simulink model "SimulinkExport"  (R2024b)
settings: Solver=FixedStepDiscrete  StartTime=0.0  StopTime=20  FixedStep=0.01  MaxStep=0.001  RelTol=1e-3
settings Model: Creator=Green Crane Testbed  LastModifiedBy=Green Crane Testbed
settings ConfigComp: PLC_TargetIDE=plcopen  PLC_MultiTBSigbuilderTimeRange=off  PLC_FoldFBCallOutputVar=off  PLC_RemoveUnusedSSMethodCallArguments=off  PLC_UseCallOutputArgSyntax=off  PLC_EnableUnsignedAndDoubleTypes=off  PLC_EnableUDTSplitting=off  PLC_MaxFieldsInUDT=500  PLC_InlineEnumCastFunction=off

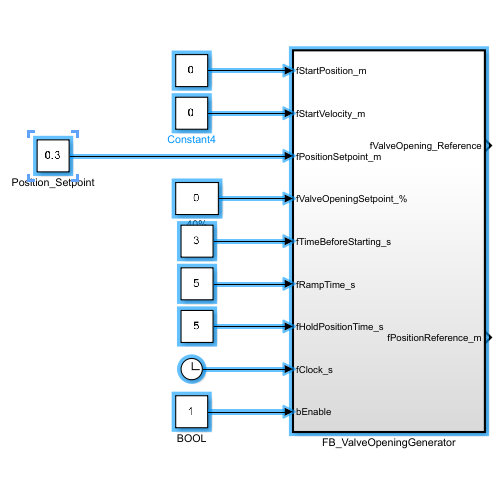
[thumbnail: Simulink's stored preview of the top-level diagram]
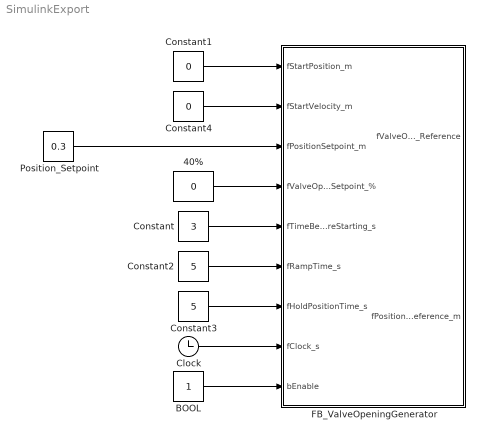
== system SimulinkExport ==
  40% : Constant  Value=0
  BOOL : Constant  OutDataTypeStr=boolean
  Clock : Clock
  Constant : Constant  Value=3
  Constant1 : Constant  Value=0
  Constant2 : Constant  Value=5
  Constant3 : Constant  Value=5
  Constant4 : Constant  Value=0
  FB_ValveOpeningGenerator : Subsystem  TreatAsAtomicUnit=on  VariantControl=Ramp_Profile
  Position_Setpoint : Constant  Value=0.3
  wires:
  40%/1 -> FB_ValveOpeningGenerator/4(fValveOpeningSetpoint_%)
  BOOL/1 -> FB_ValveOpeningGenerator/9(bEnable)
  Constant4/1 -> FB_ValveOpeningGenerator/2(fStartVelocity_m)
  Constant1/1 -> FB_ValveOpeningGenerator/1(fStartPosition_m)
  Constant2/1 -> FB_ValveOpeningGenerator/6(fRampTime_s)
  Position_Setpoint/1 -> FB_ValveOpeningGenerator/3(fPositionSetpoint_m)
  Constant3/1 -> FB_ValveOpeningGenerator/7(fHoldPositionTime_s)
  Clock/1 -> FB_ValveOpeningGenerator/8(fClock_s)
  Constant/1 -> FB_ValveOpeningGenerator/5(fTimeBeforeStarting_s)

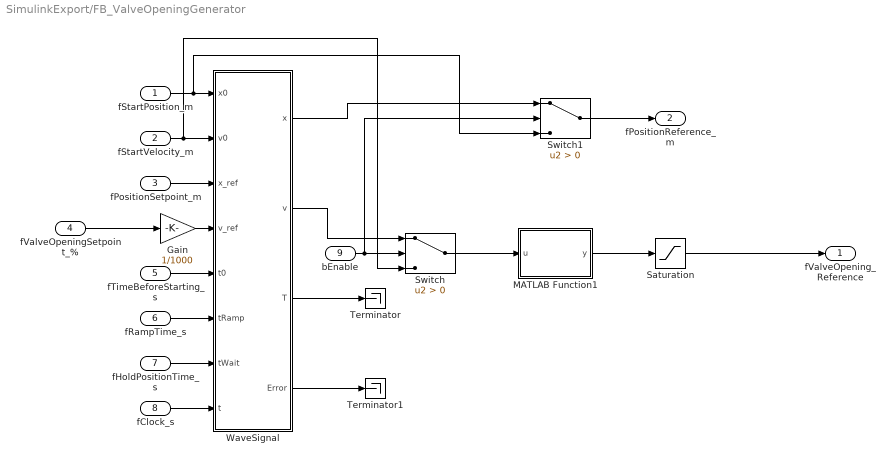
== system SimulinkExport/FB_ValveOpeningGenerator ==
  fStartPosition_m : Inport
  fStartVelocity_m : Inport  Port=2
  fPositionSetpoint_m : Inport  Port=3
  fValveOpeningSetpoint_% : Inport  Port=4
  fTimeBeforeStarting_s : Inport  Port=5
  fRampTime_s : Inport  Port=6
  fHoldPositionTime_s : Inport  Port=7
  fClock_s : Inport  Port=8
  bEnable : Inport  Port=9  OutDataTypeStr=boolean
  Gain : Gain  Gain=1/1000
  MATLAB Function1 : MATLAB Function  TreatAsAtomicUnit=on
  Saturation : Saturate
  Switch : Switch  Criteria=u2 > Threshold  SaturateOnIntegerOverflow=off  InputSameDT=off
  Switch1 : Switch  Criteria=u2 > Threshold  SaturateOnIntegerOverflow=off  InputSameDT=off
  Terminator : Terminator
  Terminator1 : Terminator
  WaveSignal : MATLAB Function  TreatAsAtomicUnit=on
  fValveOpening_Reference : Outport  VectorParamsAs1DForOutWhenUnconnected=off
  fPositionReference_m : Outport  Port=2  VectorParamsAs1DForOutWhenUnconnected=off
  wires:
  fClock_s/1 -> WaveSignal/8(t)
  fTimeBeforeStarting_s/1 -> WaveSignal/5(t0)
  fPositionSetpoint_m/1 -> WaveSignal/3(x_ref)
  fHoldPositionTime_s/1 -> WaveSignal/7(tWait)
  fValveOpeningSetpoint_%/1 -> Gain/1
  WaveSignal/3(T) -> Terminator/1
  fRampTime_s/1 -> WaveSignal/6(tRamp)
  WaveSignal/4(Error) -> Terminator1/1
  WaveSignal/2(v) -> Switch/1
  fStartPosition_m/1 -> Switch1/3, WaveSignal/1(x0)
  bEnable/1 -> Switch1/2, Switch/2
  WaveSignal/1(x) -> Switch1/1
  fStartVelocity_m/1 -> WaveSignal/2(v0), Switch/3
  MATLAB Function1/1(y) -> Saturation/1
  Switch/1 -> MATLAB Function1/1(u)
  Saturation/1 -> fValveOpening_Reference/1
  Switch1/1 -> fPositionReference_m/1
  Gain/1 -> WaveSignal/4(v_ref)

== matlab function SimulinkExport/FB_ValveOpeningGenerator/WaveSignal ==
  data: x0 input; v0 input; x_ref input; x output; v_ref input; t0 input; tRamp input; tWait input; v output; t input; T output; Error output double
function [x,v,T, Error] = fcn(x0,v0, x_ref,v_ref,t0,tRamp,tWait,t)
x_SP = x_ref - x0;
vs=v_ref;
slopeExt=v0-vs;
slopeRetr=-vs-v0;

as = vs/tRamp;
s_acc=(vs^2-v0^2)/as;

tHold=(x_SP-s_acc)/vs;

if tHold < 0
    Error = 1;
else
    Error = 0;
end

t1=tRamp;
t2=tHold;
t3=tRamp;
t4=tWait;
t5=t1;
t6=t2;
t7=t3;

x = x0;
x1 = x0 + v0*((t0+t1)-t0)-(slopeExt/t1)*((t0+t1)-t0)^2/2;
x2 = x1 + vs*((t0+t1+t2)-(t0+t1));
x4 = x_ref - v0*((t0+t1+t2+t3+t4+t5)-(t0+t1+t2+t3+t4))+(slopeRetr/t5)*((t0+t1+t2+t3+t4+t5)-(t0+t1+t2+t3+t4))^2/2;
x5 = x4-vs*((t0+t1+t2+t3+t4+t5+t6)-(t0+t1+t2+t3+t4+t5));

if Error == 1
    x = x0;
    v = v0;
elseif t>=0 && t<t0
    x = x0;
    v = v0;
elseif t>=t0 && t<(t0+t1)
    x = x0 + v0*(t-t0)-(slopeExt/t1)*(t-t0)^2/2;
    v = v0-(slopeExt/t1)*(t-t0);
elseif t>=(t0+t1) && t<(t0+t1+t2)
    x = x1 + vs*(t-(t0+t1));
    v = vs;
elseif t>=(t0+t1+t2) && t<(t0+t1+t2+t3)
    x = x2+vs*(t-(t0+t1+t2))+(slopeExt/t3)*(t-(t0+t1+t2))^2/2;
    v = vs+(slopeExt/t3)*(t-(t0+t1+t2));
elseif t>=(t0+t1+t2+t3) && t<(t0+t1+t2+t3+t4)
    x = x_ref;
    v = v0;
elseif t>=(t0+t1+t2+t3+t4) && t<(t0+t1+t2+t3+t4+t5)
    x = x_ref - v0*(t-(t0+t1+t2+t3+t4))+(slopeRetr/t5)*(t-(t0+t1+t2+t3+t4))^2/2;
    v = v0+(slopeRetr/t5)*(t-(t0+t1+t2+t3+t4));
elseif t>=(t0+t1+t2+t3+t4+t5) && t<(t0+t1+t2+t3+t4+t5+t6)
    x = x4-vs*(t-(t0+t1+t2+t3+t4+t5));
    v = -vs;
elseif t>=(t0+t1+t2+t3+t4+t5+t6) && t<(t0+t1+t2+t3+t4+t5+t6+t7)
    x = x5-vs*(t-(t0+t1+t2+t3+t4+t5+t6))-(slopeRetr/t3)*(t-(t0+t1+t2+t3+t4+t5+t6))^2/2;
    v = -vs-(slopeRetr/t3)*(t-(t0+t1+t2+t3+t4+t5+t6));
else
    x = x0;
    v = v0;
end

T = t0+t1+t2+t3+t4+t5+t6+t7;

== matlab function SimulinkExport/FB_ValveOpeningGenerator/MATLAB Function1 ==
  data: u input; y output
function y = fcn(u)



y = u/0.1;
